simulink model "InnerOuter_Sim"  (Simulink 6.6)
settings: Solver=ode4  StartTime=0.0  StopTime=700  FixedStep=SampleT  RelTol=1e-3
InitFcn:
  | clc
  | Rascal_Var
  | innerOuterInit
  | wpFile
values from neighbouring files (symbols this model uses):
  A1 = 0.007    [Rascal_Var.m]
  Apolar = 0.057    [Rascal_Var.m]
  apSampleTime = 0.01    [innerOuterInit.m]
  CD0 = 0.022    [Rascal_Var.m]
  chord = S/span    (= 0.351341681574)    [Rascal_Var.m]
  CL0 = 0.38    [Rascal_Var.m]
  CLa = 18.5    [Rascal_Var.m]
  CLa_dot = 2.64    [Rascal_Var.m]
  Clb = -0.296    [Rascal_Var.m]
  ClDa = 0.1695    [Rascal_Var.m]
  CLDe = 0.24    [Rascal_Var.m]
  CLDf = 0.4    [Rascal_Var.m]
  ClDr = 0.106    [Rascal_Var.m]
  Clp = -1.96    [Rascal_Var.m]
  CLq = 7.4    [Rascal_Var.m]
  Clr = 0.103    [Rascal_Var.m]
  Cm0 = 0.3    [Rascal_Var.m]
  Cma = -1.239    [Rascal_Var.m]
  CmDe = -3.2    [Rascal_Var.m]
  CmDf = -.021    (= -0.021)    [Rascal_Var.m]
  Cmq = -2.4    [Rascal_Var.m]
  Cnb = 0.277    [Rascal_Var.m]
  CnDa = -0.023    [Rascal_Var.m]
  CnDr = -0.1997    [Rascal_Var.m]
  Cnp = -0.0889    [Rascal_Var.m]
  Cnr = -0.19997    [Rascal_Var.m]
  CYb = -1.098    [Rascal_Var.m]
  CYDr = 0.143    [Rascal_Var.m]
  derivativesConstant = 5    [innerOuterInit.m]
  elarm = 1.21    [Rascal_Var.m]
  Euler_0 = [0; 0; 90*pi/180]'    [Rascal_Var.m]    (also in randomInit.m = double([0; 0; psi_ic]'))
  ISA_g = 9.815    [Rascal_Var.m]
  Ixx = 4.12    [Rascal_Var.m]
  Iyy = 9.58    [Rascal_Var.m]
  Izz = 9.85    [Rascal_Var.m]
  mass = 0.45359237*18    (= 8.16466266)    [Rascal_Var.m]
  MinThK = 0.077    [Rascal_Var.m]
  Pos_0 = [0; 0 ;450]'    [Rascal_Var.m]    (also in randomInit.m = double([x_ic y_ic z_ic]))
  PQR_0 = [0;0;0]'    [Rascal_Var.m]
  SampleT = 0.005    [Rascal_Var.m]    (also in innerOuterInit.m)
  span = 2.795    [Rascal_Var.m]
  ThK = 2.17    [Rascal_Var.m]
  Vb_0 = [ 25; 0;0]'    [Rascal_Var.m]
  wpCount = uint8(floor(getRanVal(7,4,10)))    [randomInit.m]
undefined symbols (not defined in the file or in its folder): bankCommandLimit, clock, daLimit, deg, deLimit, DiscIntNeverNeededParam, drLimit, dtLimit, Earth, heightErrorLimit, pitchCommandLimit, pitchErrorLimit, rad, rollControlLimit, s, uHoldLimit, WGS84, yawDamperLimit
libraries: simulink x54, SLUGS_Library x14, aerolibconvert2 x9, aerolibtransform2 x2, aerolibwind2 x1, aerolibatmos2 x1, dspmtrx3 x1, dsPICdrivers x1
(part 1 of 2)
CloseFcn:
  | rtwprivate ssgencode ModelCloseRequest AttitudeComplementary
settings Model: Creator=ASL_Lab  LastModifiedBy=Administrator
settings DebuggingCC: ConsistencyChecking=warning  AlgebraicLoopMsg=error  MultiTaskDSMMsg=warning  MultiTaskCondExecSysMsg=none  ModelReferenceExtraNoncontSigs=warning  StrictBusMsg=None
settings HardwareCC: TargetHWDeviceType=32-bit Generic
settings RTWCC: IncludeERTFirstTime=on

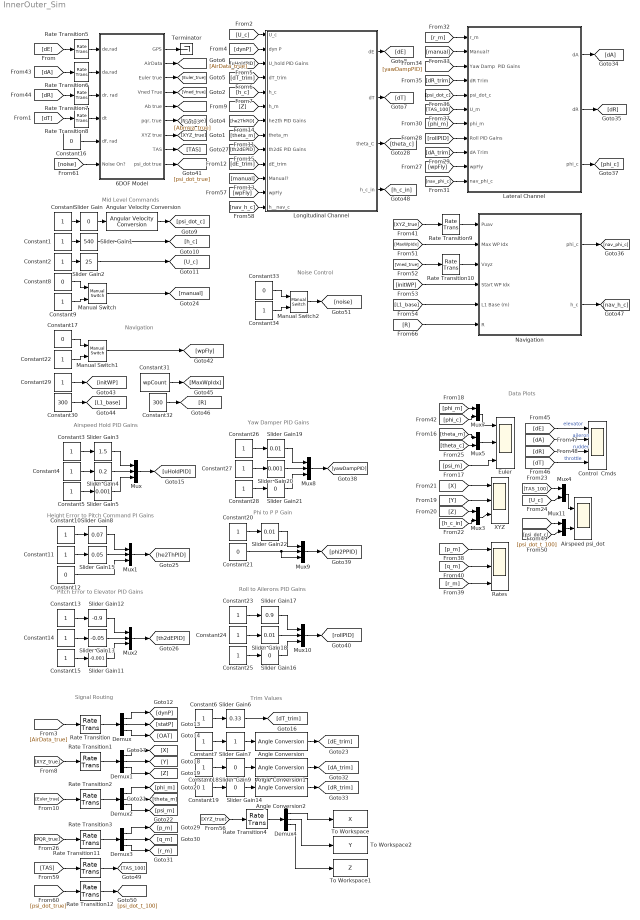
== system InnerOuter_Sim ==
  note: Mid Level Commands
  note: Trim Values
  note: Signal Routing
  note: Airspeed Hold PID Gains
  note: Height Error to Pitch Command PI Gains
  note: Pitch Error to Elevator PID Gains
  note: Data Plots
  note: Yaw Damper PID Gains
  note: Phi to P P Gain
  note: Roll to Ailerons PID Gains
  note: Navigation
  note: Noise Control
  6DOF Model : Subsystem
  Airspeed psi_dot : Scope  NumInputPorts=2
      settings: TimeRange=300  YMin=22.5~-0.3  YMax=37.5~0.25  SaveName=AirspeedPsiDot
  Angle Conversion : aerolibconvert2/Angle Conversion  SystemSampleTime=-1  IU=deg  OU=rad
  Angle Conversion1 : aerolibconvert2/Angle Conversion  SystemSampleTime=-1  IU=deg  OU=rad
  Angle Conversion2 : aerolibconvert2/Angle Conversion  SystemSampleTime=-1  IU=deg  OU=rad
  Angular Velocity Conversion : aerolibconvert2/Angular Velocity Conversion  SystemSampleTime=-1  IU=deg/s  OU=rad/s
  Constant{,1..7,9..11,13..15,18..20,22..29} (25 alike) : Constant  SampleTime=apSampleTime
  Constant{8,12,17,21} (4 alike) : Constant  Value=0  SampleTime=apSampleTime
  Constant16 : Constant  Value=0
  Constant30 : Constant  Value=300  SampleTime=apSampleTime
  Constant31 : Constant  Value=wpCount  SampleTime=apSampleTime
  Constant32 : Constant  Value=300  SampleTime=apSampleTime
  Constant33 : Constant  Value=0  SampleTime=SampleT
  Constant34 : Constant  SampleTime=SampleT
  Control  Cmds : Scope  NumInputPorts=4
      settings: TickLabels=on  TimeRange=300  YMin=-0.15~-0.075~-0.0015~0.4  YMax=0.15~0.1~0.002~0.9  SaveName=ScopeData12
  Demux{,1..4} (5 alike) : Demux  Outputs=3
  Euler : Scope  NumInputPorts=3
      settings: TimeRange=300  YMin=-0.35~-0.3~-0.5  YMax=0.7~0.3~6.5  SaveName=EulerData  DataFormat=Structure
  Lateral Channel : Subsystem  TreatAsAtomicUnit=on
  Longitudinal Channel : Subsystem  TreatAsAtomicUnit=on
  Manual Switch : simulink/Signal Routing/Manual Switch  SystemSampleTime=-1  sw=1  action=0  varsize=off
  Manual Switch1 : simulink/Signal Routing/Manual Switch  SystemSampleTime=-1  sw=0  action=0  varsize=off
  Manual Switch2 : simulink/Signal Routing/Manual Switch  SystemSampleTime=-1  sw=0  action=0  varsize=off
  Mux{,1..2,8..10} (6 alike) : Mux  Inputs=3
  Mux{3..5,7,11} (5 alike) : Mux  Inputs=2
  Navigation : Subsystem  TreatAsAtomicUnit=on
  Rate Transition{,1..4,9..12} (9 alike) : RateTransition  OutPortSampleTime=apSampleTime
  Rate Transition{5..8} (4 alike) : RateTransition  OutPortSampleTime=SampleT
  Rates : Scope  NumInputPorts=3
      settings: TimeRange=300  YMin=-0.75~-1.5~-0.3  YMax=1~1.5~0.7  SaveName=ScopeData3
  Slider Gain : simulink/Math Operations/Slider Gain  SystemSampleTime=-1  low=-20  gain=0  high=20
  Slider Gain1 : simulink/Math Operations/Slider Gain  SystemSampleTime=-1  low=0  gain=540  high=800
  Slider Gain11 : simulink/Math Operations/Slider Gain  SystemSampleTime=-1  low=-0.1  gain=-0.001  high=0
  Slider Gain12 : simulink/Math Operations/Slider Gain  SystemSampleTime=-1  low=-0.9  gain=-0.9  high=0.3
  Slider Gain13 : simulink/Math Operations/Slider Gain  SystemSampleTime=-1  low=-0.05  gain=-0.05  high=0
  Slider Gain14 : simulink/Math Operations/Slider Gain  SystemSampleTime=-1  low=-10  gain=0  high=10
  Slider Gain15 : simulink/Math Operations/Slider Gain  SystemSampleTime=-1  low=-20  gain=0.05  high=20
  Slider Gain16 : simulink/Math Operations/Slider Gain  SystemSampleTime=-1  low=-0.1  gain=0  high=0
  Slider Gain17 : simulink/Math Operations/Slider Gain  SystemSampleTime=-1  low=-0.1  gain=0.9  high=5
  Slider Gain18 : simulink/Math Operations/Slider Gain  SystemSampleTime=-1  low=-0.01  gain=0.01  high=0.01
  Slider Gain19 : simulink/Math Operations/Slider Gain  SystemSampleTime=-1  low=-20  gain=0.01  high=20
  Slider Gain2 : simulink/Math Operations/Slider Gain  SystemSampleTime=-1  low=1  gain=25  high=40
  Slider Gain20 : simulink/Math Operations/Slider Gain  SystemSampleTime=-1  low=-20  gain=0.001  high=20
  Slider Gain21 : simulink/Math Operations/Slider Gain  SystemSampleTime=-1  low=-20  gain=0  high=20
  Slider Gain22 : simulink/Math Operations/Slider Gain  SystemSampleTime=-1  low=-20  gain=0.01  high=20
  Slider Gain3 : simulink/Math Operations/Slider Gain  SystemSampleTime=-1  low=-20  gain=1.5  high=20
  Slider Gain4 : simulink/Math Operations/Slider Gain  SystemSampleTime=-1  low=-20  gain=0.2  high=20
  Slider Gain5 : simulink/Math Operations/Slider Gain  SystemSampleTime=-1  low=-20  gain=0.001  high=20
  Slider Gain6 : simulink/Math Operations/Slider Gain  SystemSampleTime=-1  low=0.1  gain=0.33  high=1
  Slider Gain7 : simulink/Math Operations/Slider Gain  SystemSampleTime=-1  low=-10  gain=1  high=10
  Slider Gain8 : simulink/Math Operations/Slider Gain  SystemSampleTime=-1  low=-20  gain=0.07  high=20
  Slider Gain9 : simulink/Math Operations/Slider Gain  SystemSampleTime=-1  low=-10  gain=0  high=10
  Terminator : Terminator
  To Workspace : ToWorkspace  VariableName=X  SampleTime=-1  SaveFormat=Array
  To Workspace1 : ToWorkspace  VariableName=Z  SampleTime=-1  SaveFormat=Array
  To Workspace2 : ToWorkspace  VariableName=Y  SampleTime=-1  SaveFormat=Array
  XYZ : Scope  NumInputPorts=3
      settings: TimeRange=300  YMin=0~-400~0  YMax=2500~700~800
  wires:
  6DOF Model/7(XYZ true) -> [XYZ_true]
  6DOF Model/4(Vned True) -> [Vned_true]
  6DOF Model/5(Ab true) -> [Abmea_true]
  6DOF Model/6("pqr, true") -> [PQR_true]
  6DOF Model/3(Euler true) -> [Euler_true]
  6DOF Model/2(AirData) -> [AirData_true]
  Longitudinal Channel/1(dE) -> [dE]
  Longitudinal Channel/2(dT) -> [dT]
  Constant/1 -> Slider Gain/1
  Constant1/1 -> Slider Gain1/1
  Constant2/1 -> Slider Gain2/1
  Slider Gain/1 -> Angular Velocity Conversion/1
  Angular Velocity Conversion/1 -> [psi_dot_c]
  Slider Gain2/1 -> [U_c]
  [U_c] -> Longitudinal Channel/1(U_c)
  [AirData_true] -> Rate Transition/1
  Demux/1 -> [dynP]
  Demux/2 -> [statP]
  Demux/3 -> [OAT]
  Constant3/1 -> Slider Gain3/1
  Constant4/1 -> Slider Gain4/1
  Constant5/1 -> Slider Gain5/1
  Slider Gain4/1 -> Mux/2
  Slider Gain3/1 -> Mux/1
  Slider Gain5/1 -> Mux/3
  Mux/1 -> [uHoldPID]
  [dynP] -> Longitudinal Channel/2(dyn P)
  [uHoldPID] -> Longitudinal Channel/3(U_hold PID Gains)
  Constant6/1 -> Slider Gain6/1
  Slider Gain6/1 -> [dT_trim]
  [dT_trim] -> Longitudinal Channel/4(dT_trim)
  [h_c] -> Longitudinal Channel/5(h_c)
  [XYZ_true] -> Rate Transition1/1
  Demux1/1 -> [X]
  Demux1/2 -> [Y]
  Demux1/3 -> [Z]
  [Z] -> Longitudinal Channel/6(h_m)
  [Euler_true] -> Rate Transition2/1
  Demux2/1 -> [phi_m]
  Demux2/2 -> [theta_m]
  Demux2/3 -> [psi_m]
  [theta_m] -> Longitudinal Channel/8(theta_m)
  Constant7/1 -> Slider Gain7/1
  Slider Gain7/1 -> Angle Conversion/1
  Angle Conversion/1 -> [dE_trim]
  [dE_trim] -> Longitudinal Channel/10(dE_trim)
  Constant8/1 -> Manual Switch/1
  Constant9/1 -> Manual Switch/2
  Manual Switch/1 -> [manual]
  [manual] -> Longitudinal Channel/11(Manual?)
  Constant10/1 -> Slider Gain8/1
  Constant11/1 -> Slider Gain15/1
  Constant12/1 -> Mux1/3
  Slider Gain8/1 -> Mux1/1
  Mux1/1 -> [he2ThPID]
  Constant13/1 -> Slider Gain12/1
  Constant14/1 -> Slider Gain13/1
  Constant15/1 -> Slider Gain11/1
  Slider Gain13/1 -> Mux2/2
  Slider Gain12/1 -> Mux2/1
  Slider Gain11/1 -> Mux2/3
  Mux2/1 -> [th2dEPID]
  [he2ThPID] -> Longitudinal Channel/7(he2th PID Gains)
  [th2dEPID] -> Longitudinal Channel/9(th2dE PID Gains)
  Mux5/1 -> Euler/2
  [psi_m] -> Euler/3
  [X] -> XYZ/1
  [Y] -> XYZ/2
  Mux3/1 -> XYZ/3
  [Z] -> Mux3/1
  [h_c_in] -> Mux3/2
  [dT] -> Rate Transition8/1
  [dE] -> Rate Transition5/1
  Mux4/1 -> Airspeed psi_dot/1
  6DOF Model/8(TAS) -> [TAS]
  [TAS_100] -> Mux4/1
  [U_c] -> Mux4/2
  [theta_c] -> Mux5/2
  Longitudinal Channel/3(theta_C) -> [theta_c]
  [PQR_true] -> Rate Transition3/1
  Demux3/1 -> [p_m]
  Demux3/2 -> [q_m]
  Demux3/3 -> [r_m]
  Constant18/1 -> Slider Gain9/1
  Slider Gain9/1 -> Angle Conversion1/1
  Angle Conversion1/1 -> [dA_trim]
  Constant19/1 -> Slider Gain14/1
  Slider Gain14/1 -> Angle Conversion2/1
  Angle Conversion2/1 -> [dR_trim]
  [r_m] -> Lateral Channel/1(r_m)
  [manual] -> Lateral Channel/2(Manual?)
  [yawDampPID] -> Lateral Channel/3(Yaw Damp  PID Gains)
  [dR_trim] -> Lateral Channel/4(dR Trim)
  [psi_dot_c] -> Lateral Channel/5(psi_dot_c)
  [TAS_100] -> Lateral Channel/6(U_m)
  [phi_m] -> Lateral Channel/7(phi_m)
  [rollPID] -> Lateral Channel/8(Roll PID Gains)
  [dA_trim] -> Lateral Channel/9(dA Trim)
  [r_m] -> Rates/3
  Lateral Channel/1(dA) -> [dA]
  Lateral Channel/2(dR) -> [dR]
  Lateral Channel/3(phi_c) -> [phi_c]
  [q_m] -> Rates/2
  [phi_m] -> Mux7/1
  [phi_c] -> Mux7/2
  Mux7/1 -> Euler/1
  Constant26/1 -> Slider Gain19/1
  Constant27/1 -> Slider Gain20/1
  Constant28/1 -> Slider Gain21/1
  Slider Gain20/1 -> Mux8/2
  Slider Gain19/1 -> Mux8/1
  Slider Gain21/1 -> Mux8/3
  Mux8/1 -> [yawDampPID]
  Constant20/1 -> Slider Gain22/1
  Constant21/1 -> Mux9/2, Mux9/3
  Slider Gain22/1 -> Mux9/1
  Mux9/1 -> [phi2PPID]
  Constant23/1 -> Slider Gain17/1
  Constant24/1 -> Slider Gain18/1
  Constant25/1 -> Slider Gain16/1
  Slider Gain18/1 -> Mux10/2
  Slider Gain17/1 -> Mux10/1
  Slider Gain16/1 -> Mux10/3
  Mux10/1 -> [rollPID]
  [dA] -> Rate Transition6/1
  [dR] -> Rate Transition7/1
  Constant16/1 -> 6DOF Model/5("df, rad")
  Slider Gain15/1 -> Mux1/2
  [dE] -> Control  Cmds/1  "elevator"
  [dA] -> Control  Cmds/2  "aileron"
  [dR] -> Control  Cmds/3  "rudder"
  [dT] -> Control  Cmds/4  "throttle"
  [theta_m] -> Mux5/1
  6DOF Model/9(psi_dot true) -> [psi_dot_true]
  [psi_dot_t_100] -> Mux11/1
  [psi_dot_c] -> Mux11/2
  Mux11/1 -> Airspeed psi_dot/2
  [p_m] -> Rates/1
  Constant17/1 -> Manual Switch1/1
  Constant22/1 -> Manual Switch1/2
  Manual Switch1/1 -> [wpFly]
  Constant29/1 -> [initWP]
  Slider Gain1/1 -> [h_c]
  [wpFly] -> Lateral Channel/10(wpFly)
  Navigation/1(phi_c) -> [nav_phi_c]
  [nav_phi_c] -> Lateral Channel/11(nav_phi_c)
  [XYZ_true] -> Rate Transition9/1
  Constant30/1 -> [L1_base]
  Constant31/1 -> [MaxWpIdx]
  [MaxWpIdx] -> Navigation/2(Max WP Idx)
  [Vned_true] -> Rate Transition10/1
  [initWP] -> Navigation/4(Start WP Idx)
  [L1_base] -> Navigation/5(L1 Base (m))
  [XYZ_true] -> Rate Transition4/1
  Demux4/1 -> To Workspace/1
  Demux4/2 -> To Workspace2/1
  Demux4/3 -> To Workspace1/1
  Navigation/2(h_c) -> [nav_h_c]
  [wpFly] -> Longitudinal Channel/12(wpFly)
  [nav_h_c] -> Longitudinal Channel/13(h__nav_c)
  Longitudinal Channel/4(h_c_in) -> [h_c_in]
  Rate Transition/1 -> Demux/1
  Rate Transition1/1 -> Demux1/1
  Rate Transition2/1 -> Demux2/1
  Rate Transition3/1 -> Demux3/1
  Rate Transition4/1 -> Demux4/1
  Rate Transition5/1 -> 6DOF Model/1(de,rad)
  Rate Transition6/1 -> 6DOF Model/2(da,rad)
  Rate Transition7/1 -> 6DOF Model/3("dr, rad")
  Rate Transition8/1 -> 6DOF Model/4(dt)
  Rate Transition9/1 -> Navigation/1(Puav)
  Rate Transition10/1 -> Navigation/3(Vxyz)
  [TAS] -> Rate Transition11/1
  Rate Transition11/1 -> [TAS_100]
  [psi_dot_true] -> Rate Transition12/1
  Rate Transition12/1 -> [psi_dot_t_100]
  Constant33/1 -> Manual Switch2/1
  Constant34/1 -> Manual Switch2/2
  Manual Switch2/1 -> [noise]
  [noise] -> 6DOF Model/6(Noise On?)
  Constant32/1 -> [R]
  [R] -> Navigation/6(R)
  6DOF Model/1(GPS) -> Terminator/1

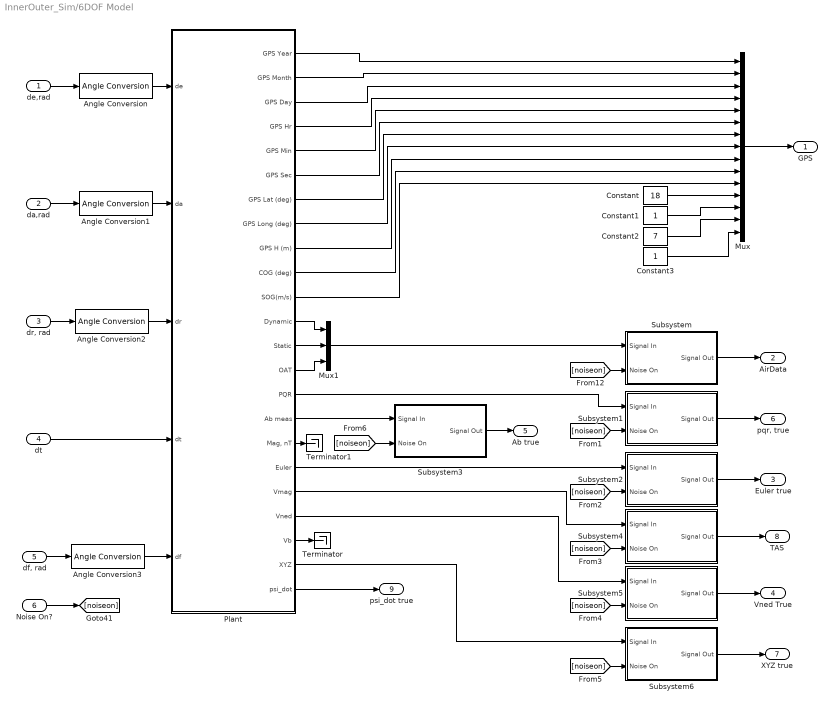
== system InnerOuter_Sim/6DOF Model ==
  de,rad : Inport
  da,rad : Inport  Port=2
  "dr, rad" : Inport  Port=3
  dt : Inport  Port=4
  "df, rad" : Inport  Port=5
  Noise On? : Inport  Port=6
  Angle Conversion{,1..3} (4 alike) : aerolibconvert2/Angle Conversion  SystemSampleTime=-1  IU=rad  OU=deg
  Constant : Constant  Value=18  SampleTime=SampleT
  Constant1 : Constant  SampleTime=SampleT
  Constant2 : Constant  Value=7  SampleTime=SampleT
  Constant3 : Constant  SampleTime=SampleT
  Mux : Mux  Inputs=15
  Mux1 : Mux  Inputs=3
  Plant : Subsystem
  Subsystem : Subsystem  mask{nv=[0.01 0.01 0.1], st=SampleT, ns=[132 564 987]}
      mask prompts: nv "Noise Variance"; st "Sample Time"; ns "Noise Seed"
  Subsystem1 : Subsystem  mask{nv=[0.001 0.001 0.001], st=SampleT, ns=[132 564 987]}
      mask prompts: nv "Noise Variance"; st "Sample Time"; ns "Noise Seed"
  Subsystem2 : Subsystem  mask{nv=[0.0001 0.00003 0.0001], st=SampleT, ns=[132 564 987]}
      mask prompts: nv "Noise Variance"; st "Sample Time"; ns "Noise Seed"
  Subsystem3 : Subsystem  mask{nv=[0.1 0.1 0.1], st=SampleT, ns=[132 564 987]}
      mask prompts: nv "Noise Variance"; st "Sample Time"; ns "Noise Seed"
  Subsystem4 : Subsystem  mask{nv=[0.01], st=SampleT, ns=[321564]}
      mask prompts: nv "Noise Variance"; st "Sample Time"; ns "Noise Seed"
  Subsystem5 : Subsystem  mask{nv=[0.01 0.01 0.01], st=SampleT, ns=[321564 6546 98798]}
      mask prompts: nv "Noise Variance"; st "Sample Time"; ns "Noise Seed"
  Subsystem6 : Subsystem  mask{nv=[0.03 0.03 0.05], st=SampleT, ns=[321564]}
      mask prompts: nv "Noise Variance"; st "Sample Time"; ns "Noise Seed"
  Terminator : Terminator
  Terminator1 : Terminator
  GPS : Outport
  AirData : Outport  Port=2
  Euler true : Outport  Port=3
  Vned True : Outport  Port=4
  Ab true : Outport  Port=5
  "pqr, true" : Outport  Port=6
  XYZ true : Outport  Port=7
  TAS : Outport  Port=8
  psi_dot true : Outport  Port=9
  wires:
  de,rad/1 -> Angle Conversion/1
  da,rad/1 -> Angle Conversion1/1
  "dr, rad"/1 -> Angle Conversion2/1
  dt/1 -> Plant/4(dt)
  "df, rad"/1 -> Angle Conversion3/1
  Angle Conversion/1 -> Plant/1(de)
  Angle Conversion1/1 -> Plant/2(da)
  Angle Conversion2/1 -> Plant/3(dr)
  Angle Conversion3/1 -> Plant/5(df)
  Mux/1 -> GPS/1
  Plant/1(GPS Year) -> Mux/1
  Plant/2(GPS Month) -> Mux/2
  Plant/3(GPS Day) -> Mux/3
  Plant/4(GPS Hr) -> Mux/4
  Plant/5(GPS Min) -> Mux/5
  Plant/6(GPS Sec) -> Mux/6
  Plant/7(GPS Lat (deg)) -> Mux/7
  Plant/8(GPS Long (deg)) -> Mux/8
  Plant/9(GPS H (m)) -> Mux/9
  Plant/10(COG (deg)) -> Mux/10
  Plant/11(SOG(m/s)) -> Mux/11
  Plant/12(Dynamic) -> Mux1/1
  Plant/13(Static) -> Mux1/2
  Plant/14(OAT) -> Mux1/3
  Mux1/1 -> Subsystem/1(Signal In)
  Constant/1 -> Mux/12
  Constant1/1 -> Mux/13
  Constant2/1 -> Mux/14
  Constant3/1 -> Mux/15
  Plant/23(psi_dot) -> psi_dot true/1
  Noise On?/1 -> [noiseon]
  Subsystem/1(Signal Out) -> AirData/1
  [noiseon] -> Subsystem/2(Noise On)
  [noiseon] -> Subsystem1/2(Noise On)
  [noiseon] -> Subsystem2/2(Noise On)
  [noiseon] -> Subsystem4/2(Noise On)
  [noiseon] -> Subsystem5/2(Noise On)
  [noiseon] -> Subsystem6/2(Noise On)
  [noiseon] -> Subsystem3/2(Noise On)
  Subsystem1/1(Signal Out) -> "pqr, true"/1
  Plant/15(PQR) -> Subsystem1/1(Signal In)
  Subsystem2/1(Signal Out) -> Euler true/1
  Plant/18(Euler) -> Subsystem2/1(Signal In)
  Subsystem3/1(Signal Out) -> Ab true/1
  Plant/16(Ab meas) -> Subsystem3/1(Signal In)
  Subsystem4/1(Signal Out) -> TAS/1
  Plant/19(Vmag) -> Subsystem4/1(Signal In)
  Subsystem5/1(Signal Out) -> Vned True/1
  Plant/20(Vned) -> Subsystem5/1(Signal In)
  Subsystem6/1(Signal Out) -> XYZ true/1
  Plant/22(XYZ) -> Subsystem6/1(Signal In)
  Plant/21(Vb) -> Terminator/1
  Plant/17("Mag, nT") -> Terminator1/1

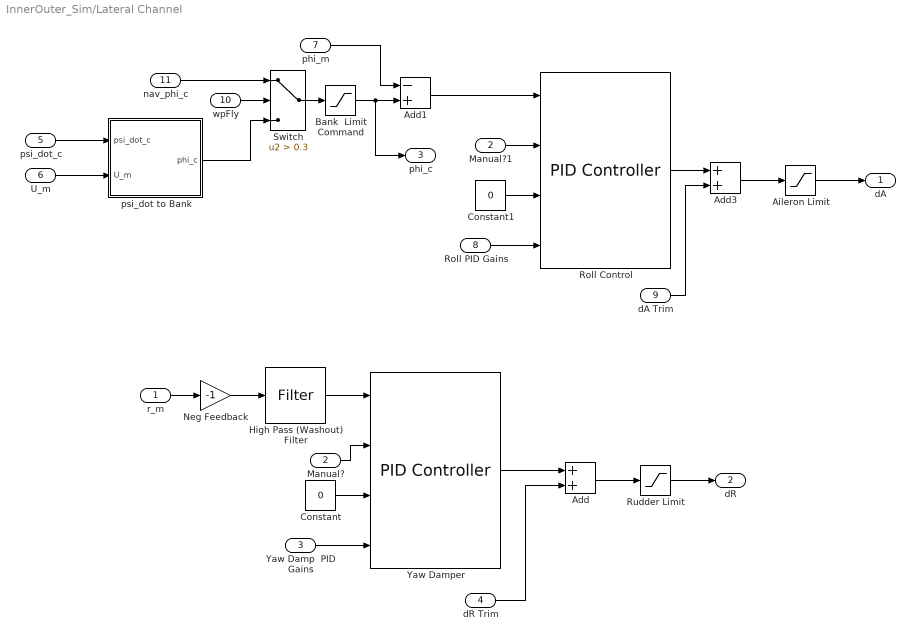
== system InnerOuter_Sim/Lateral Channel ==
  r_m : Inport
  Manual? : Inport  Port=2
  Yaw Damp  PID Gains : Inport  Port=3
  dR Trim : Inport  Port=4
  psi_dot_c : Inport  Port=5
  U_m : Inport  Port=6
  phi_m : Inport  Port=7
  Roll PID Gains : Inport  Port=8
  dA Trim : Inport  Port=9
  wpFly : Inport  Port=10  SampleTime=apSampleTime
  nav_phi_c : Inport  Port=11
  Add : Sum  OutScaling=2^-10
  Add1 : Sum  Inputs=-+  OutScaling=2^-10
  Add3 : Sum  OutScaling=2^-10
  Aileron Limit : Saturate  UpperLimit=daLimit  LowerLimit=-daLimit  SampleTime=apSampleTime
  Bank  Limit Command : Saturate  UpperLimit=bankCommandLimit  LowerLimit=-bankCommandLimit  SampleTime=apSampleTime
  Constant : Constant  Value=0
  Constant1 : Constant  Value=0
  High Pass (Washout) Filter : SLUGS_Library/Singnal Routing & Conditioning/Filter  SystemSampleTime=-1  Zeros=[0]  Poles=[-1/5]  Gain=1  AbsTol=auto  SampleTime=apSampleTime  method=tustin  Wc=1
  Manual?1 : InportShadow  Port=2  LatchByCopyingInsideSignal=off
  Neg Feedback : Gain  Gain=-1
  Roll Control : SLUGS_Library/Control Blocks/PID Controller  SystemSampleTime=-1  TSample=apSampleTime  NDelay=derivativesConstant  upperLimit=rollControlLimit  lowerLimit=-rollControlLimit
  Rudder Limit : Saturate  UpperLimit=apSampleTime  LowerLimit=-drLimit  SampleTime=apSampleTime
  Switch : Switch  Criteria=u2 > Threshold  Threshold=0.3
  Yaw Damper : SLUGS_Library/Control Blocks/PID Controller  SystemSampleTime=-1  TSample=apSampleTime  NDelay=derivativesConstant  upperLimit=yawDamperLimit  lowerLimit=-yawDamperLimit
  psi_dot to Bank : Subsystem
  dA : Outport
  dR : Outport  Port=2
  phi_c : Outport  Port=3
  wires:
  High Pass (Washout) Filter/1 -> Yaw Damper/1
  Neg Feedback/1 -> High Pass (Washout) Filter/1
  r_m/1 -> Neg Feedback/1
  Rudder Limit/1 -> dR/1
  Constant/1 -> Yaw Damper/3
  Manual?/1 -> Yaw Damper/2
  Yaw Damp  PID Gains/1 -> Yaw Damper/4
  Add/1 -> Rudder Limit/1
  Yaw Damper/1 -> Add/1
  dR Trim/1 -> Add/2
  psi_dot_c/1 -> psi_dot to Bank/1(psi_dot_c)
  U_m/1 -> psi_dot to Bank/2(U_m)
  Manual?1/1 -> Roll Control/2
  Constant1/1 -> Roll Control/3
  Roll PID Gains/1 -> Roll Control/4
  Add3/1 -> Aileron Limit/1
  Roll Control/1 -> Add3/1
  dA Trim/1 -> Add3/2
  Aileron Limit/1 -> dA/1
  Add1/1 -> Roll Control/1
  phi_m/1 -> Add1/1
  Switch/1 -> Bank  Limit Command/1
  nav_phi_c/1 -> Switch/1
  wpFly/1 -> Switch/2
  psi_dot to Bank/1(phi_c) -> Switch/3
  Bank  Limit Command/1 -> Add1/2, phi_c/1

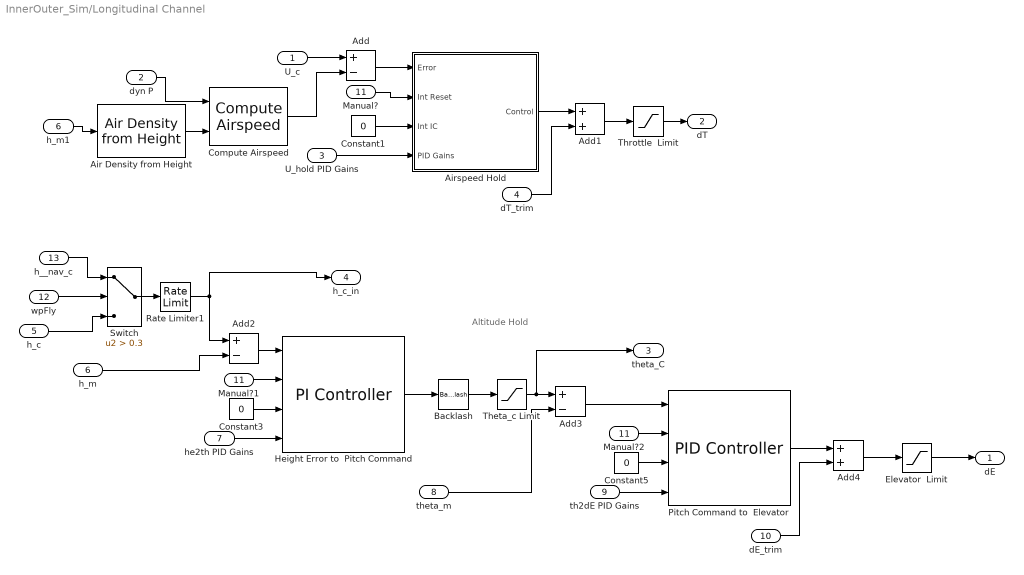
== system InnerOuter_Sim/Longitudinal Channel ==
  note: Altitude Hold
  U_c : Inport
  dyn P : Inport  Port=2
  U_hold PID Gains : Inport  Port=3
  dT_trim : Inport  Port=4
  h_c : Inport  Port=5
  h_m : Inport  Port=6
  he2th PID Gains : Inport  Port=7
  theta_m : Inport  Port=8
  th2dE PID Gains : Inport  Port=9
  dE_trim : Inport  Port=10
  Manual? : Inport  Port=11
  wpFly : Inport  Port=12  SampleTime=apSampleTime
  h__nav_c : Inport  Port=13
  Add : Sum  Inputs=+-  OutScaling=2^-10
  Add1 : Sum  Inputs=2  OutScaling=2^-10
  Add2 : Sum  Inputs=+-  OutScaling=2^-10
  Add3 : Sum  Inputs=+-  OutScaling=2^-10
  Add4 : Sum  Inputs=2  OutScaling=2^-10
  Air Density from Height : SLUGS_Library/Air Density from Height  SystemSampleTime=-1
  Airspeed Hold : Subsystem  AncestorBlock=SLUGS_Library/Control Blocks/PID Controller  mask{TSample=apSampleTime, NDelay=derivativesConstant, upperLimit=uHoldLimit, lowerLimit=0.1}
      mask prompts: TSample "Sample Time"; NDelay "Derivation Time Constant Factor (1->10)"; upperLimit "Integrator Upper Windup Limit"; lowerLimit "Integrator Lower Windup Limit"
      mask help:
      | This Block implements a PID Controller with the Following Characteristcs:
      |
      | 1.- Integrator antiwindup is given by the limits in the block
      | 2.- The time Derivative is "low-passed" by using the previous N samples instead of the one before
      | 3.- It contains an Integrator Reset if needed
  Backlash : Backlash  BacklashWidth=0.05
  Compute Airspeed : SLUGS_Library/Compute Airspeed  SystemSampleTime=-1
  Constant1 : Constant  Value=0
  Constant3 : Constant  Value=0
  Constant5 : Constant  Value=0
  Elevator  Limit : Saturate  UpperLimit=deLimit  LowerLimit=-deLimit  SampleTime=apSampleTime
  Height Error to  Pitch Command : SLUGS_Library/Control Blocks/PI Controller  SystemSampleTime=-1  TSample=apSampleTime  upperLimit=heightErrorLimit  lowerLimit=-heightErrorLimit
  Manual?1 : InportShadow  Port=11  LatchByCopyingInsideSignal=off
  Manual?2 : InportShadow  Port=11  LatchByCopyingInsideSignal=off
  Pitch Command to  Elevator : SLUGS_Library/Control Blocks/PID Controller  SystemSampleTime=-1  TSample=apSampleTime  NDelay=derivativesConstant  upperLimit=pitchErrorLimit  lowerLimit=-pitchErrorLimit
  Rate Limiter1 : RateLimiter  RisingSlewLimit=10  FallingSlewLimit=-10  SampleTimeMode=inherited
  Switch : Switch  Criteria=u2 > Threshold  Threshold=0.3
  Theta_c Limit : Saturate  UpperLimit=pitchCommandLimit  LowerLimit=-pitchCommandLimit  SampleTime=apSampleTime
  Throttle  Limit : Saturate  UpperLimit=dtLimit  LowerLimit=0  SampleTime=apSampleTime
  h_m1 : InportShadow  Port=6  LatchByCopyingInsideSignal=off
  dE : Outport
  dT : Outport  Port=2
  theta_C : Outport  Port=3
  h_c_in : Outport  Port=4
  wires:
  U_c/1 -> Add/1
  Compute Airspeed/1 -> Add/2
  Add/1 -> Airspeed Hold/1(Error)
  Airspeed Hold/1(Control) -> Add1/1
  dT_trim/1 -> Add1/2
  Add1/1 -> Throttle  Limit/1
  Constant1/1 -> Airspeed Hold/3(Int IC)
  U_hold PID Gains/1 -> Airspeed Hold/4(PID Gains)
  Throttle  Limit/1 -> dT/1
  Add2/1 -> Height Error to  Pitch Command/1
  h_m/1 -> Add2/2
  Constant3/1 -> Height Error to  Pitch Command/3
  theta_m/1 -> Add3/2
  Constant5/1 -> Pitch Command to  Elevator/3
  Manual?/1 -> Airspeed Hold/2(Int Reset)
  Manual?1/1 -> Height Error to  Pitch Command/2
  Manual?2/1 -> Pitch Command to  Elevator/2
  Add4/1 -> Elevator  Limit/1
  Pitch Command to  Elevator/1 -> Add4/1
  dE_trim/1 -> Add4/2
  Elevator  Limit/1 -> dE/1
  Air Density from Height/1 -> Compute Airspeed/2
  dyn P/1 -> Compute Airspeed/1
  h_m1/1 -> Air Density from Height/1
  he2th PID Gains/1 -> Height Error to  Pitch Command/4
  th2dE PID Gains/1 -> Pitch Command to  Elevator/4
  Add3/1 -> Pitch Command to  Elevator/1
  Theta_c Limit/1 -> Add3/1, theta_C/1
  wpFly/1 -> Switch/2
  Switch/1 -> Rate Limiter1/1
  h_c/1 -> Switch/3
  h__nav_c/1 -> Switch/1
  Rate Limiter1/1 -> Add2/1, h_c_in/1
  Height Error to  Pitch Command/1 -> Backlash/1
  Backlash/1 -> Theta_c Limit/1

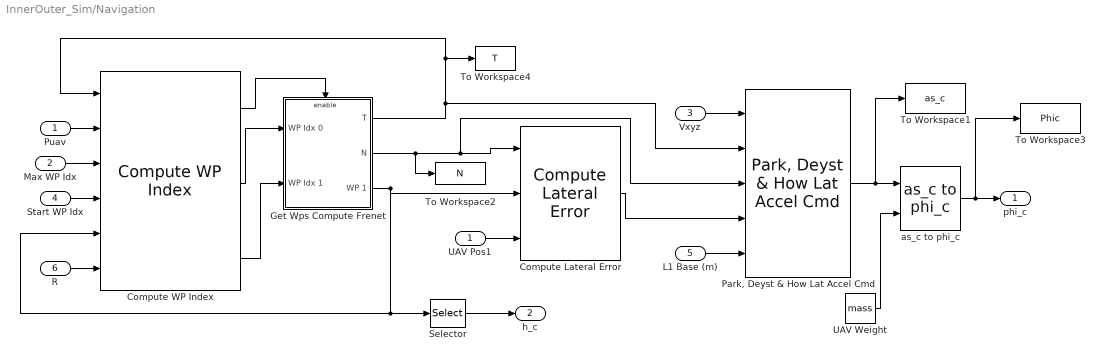
== system InnerOuter_Sim/Navigation ==
  Puav : Inport  SampleTime=apSampleTime
  Max WP Idx : Inport  Port=2
  Vxyz : Inport  Port=3
  Start WP Idx : Inport  Port=4
  L1 Base (m) : Inport  Port=5
  R : Inport  Port=6
  Compute Lateral Error : SLUGS_Library/Navigation/Compute Lateral Error  SystemSampleTime=-1
  Compute WP Index : SLUGS_Library/Navigation/Compute WP Index  SystemSampleTime=-1
  Get Wps Compute Frenet : Subsystem
  "Park, Deyst & How Lat Accel Cmd" : SLUGS_Library/Navigation/Park, Deyst & How Lat Accel Cmd  SystemSampleTime=-1
  Selector : Selector  IndexOptions=Index vector (dialog)  Indices=[3]  OutputSizes=1  InputPortWidth=3
  To Workspace1 : ToWorkspace  VariableName=as_c  SampleTime=-1  SaveFormat=Array
  To Workspace2 : ToWorkspace  VariableName=N  SampleTime=-1  SaveFormat=Array
  To Workspace3 : ToWorkspace  VariableName=Phic  SampleTime=-1  SaveFormat=Array
  To Workspace4 : ToWorkspace  VariableName=T  SampleTime=-1  SaveFormat=Array
  UAV Weight : Constant  Value=mass
  UAV Pos1 : InportShadow  Port=1  SampleTime=apSampleTime  LatchByCopyingInsideSignal=off
  as_c to phi_c : SLUGS_Library/Navigation/as_c to phi_c  SystemSampleTime=-1
  phi_c : Outport
  h_c : Outport  Port=2
  wires:
  Compute WP Index/2 -> Get Wps Compute Frenet/1(WP Idx 0)
  Compute WP Index/3 -> Get Wps Compute Frenet/2(WP Idx 1)
  Get Wps Compute Frenet/2(N) -> Compute Lateral Error/1, "Park, Deyst & How Lat Accel Cmd"/3, To Workspace2/1
  Get Wps Compute Frenet/1(T) -> To Workspace4/1, Compute WP Index/1, "Park, Deyst & How Lat Accel Cmd"/2
  Puav/1 -> Compute WP Index/2
  Max WP Idx/1 -> Compute WP Index/3
  Start WP Idx/1 -> Compute WP Index/4
  "Park, Deyst & How Lat Accel Cmd"/1 -> as_c to phi_c/1, To Workspace1/1
  UAV Pos1/1 -> Compute Lateral Error/3
  as_c to phi_c/1 -> phi_c/1, To Workspace3/1
  UAV Weight/1 -> as_c to phi_c/2
  Compute Lateral Error/1 -> "Park, Deyst & How Lat Accel Cmd"/4
  Get Wps Compute Frenet/3(WP 1) -> Compute Lateral Error/2, Selector/1, Compute WP Index/5
  Selector/1 -> h_c/1
  L1 Base (m)/1 -> "Park, Deyst & How Lat Accel Cmd"/5
  Compute WP Index/1 -> Get Wps Compute Frenet/Enable
  R/1 -> Compute WP Index/6
  Vxyz/1 -> "Park, Deyst & How Lat Accel Cmd"/1

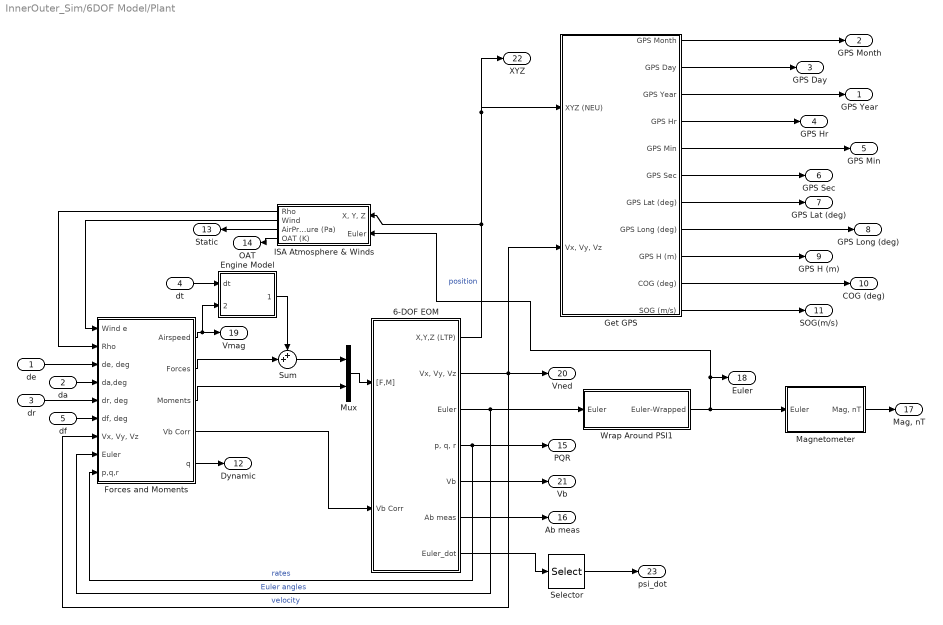
== system InnerOuter_Sim/6DOF Model/Plant ==
  de : Inport
  da : Inport  Port=2
  dr : Inport  Port=3
  dt : Inport  Port=4
  df : Inport  Port=5
  6-DOF EOM : Subsystem
  Engine Model : Subsystem
  Forces and Moments : Subsystem
  Get GPS : Subsystem
  ISA Atmosphere & Winds : Subsystem  Orientation=left
  Magnetometer : Subsystem  mask{magField=[ 23143.6 5858.2 45511.9]}
      mask prompts: magField "Local Magnetic Field"
      mask help:
      | Simulates the Data from magnetometers with no noise.
      |
      | You can obtain data for the local magnetic field at:
      |
      | http://www.ngdc.noaa.gov/geomagmodels/IGRFWMM.jsp
  Mux : Mux  Inputs=2
  Selector : Selector  IndexOptions=Index vector (dialog)  Indices=[3]  OutputSizes=1  InputPortWidth=3
  Sum : Sum  Inputs=++|  SaturateOnIntegerOverflow=on
  Wrap Around PSI1 : Subsystem
  GPS Year : Outport
  GPS Month : Outport  Port=2
  GPS Day : Outport  Port=3
  GPS Hr : Outport  Port=4
  GPS Min : Outport  Port=5
  GPS Sec : Outport  Port=6
  GPS Lat (deg) : Outport  Port=7
  GPS Long (deg) : Outport  Port=8
  GPS H (m) : Outport  Port=9
  COG (deg) : Outport  Port=10
  SOG(m/s) : Outport  Port=11
  Dynamic : Outport  Port=12
  Static : Outport  Orientation=left  Port=13
  OAT : Outport  Orientation=left  Port=14
  PQR : Outport  Port=15
  Ab meas : Outport  Port=16
  "Mag, nT" : Outport  Port=17
  Euler : Outport  Port=18
  Vmag : Outport  Port=19
  Vned : Outport  Port=20
  Vb : Outport  Port=21
  XYZ : Outport  Port=22
  psi_dot : Outport  Port=23
  wires:
  Get GPS/1(GPS Month) -> GPS Month/1
  Get GPS/2(GPS Day) -> GPS Day/1
  Get GPS/3(GPS Year) -> GPS Year/1
  Get GPS/4(GPS Hr) -> GPS Hr/1
  Get GPS/5(GPS Min) -> GPS Min/1
  Get GPS/6(GPS Sec) -> GPS Sec/1
  Get GPS/7(GPS Lat (deg)) -> GPS Lat (deg)/1
  Get GPS/8(GPS Long (deg)) -> GPS Long (deg)/1
  Get GPS/9(GPS H (m)) -> GPS H (m)/1
  6-DOF EOM/6(Ab meas) -> Ab meas/1
  Mux/1 -> 6-DOF EOM/1("[F,M]")
  6-DOF EOM/5(Vb) -> Vb/1
  Engine Model/1(Thrust) -> Sum/1
  Forces and Moments/5(q) -> Dynamic/1
  ISA Atmosphere & Winds/3(AirPressure (Pa)) -> Static/1
  Forces and Moments/1(Airspeed) -> Engine Model/2(Vmag), Vmag/1
  ISA Atmosphere & Winds/2(Wind) -> Forces and Moments/1(Wind e)
  ISA Atmosphere & Winds/1(Rho) -> Forces and Moments/2(Rho)
  Forces and Moments/3(Moments) -> Mux/2
  Forces and Moments/2(Forces) -> Sum/2
  Sum/1 -> Mux/1
  Forces and Moments/4(Vb Corr) -> 6-DOF EOM/2(Vb Corr)
  6-DOF EOM/1(X,Y,Z (LTP)) -> ISA Atmosphere & Winds/1("X, Y, Z"), Get GPS/1(XYZ (NEU)), XYZ/1  "position"
  6-DOF EOM/2("Vx, Vy, Vz") -> Vned/1, Get GPS/2("Vx, Vy, Vz"), Forces and Moments/7("Vx, Vy, Vz ")  "velocity"
  6-DOF EOM/3(Euler) -> Wrap Around PSI1/1(Euler), Forces and Moments/8(Euler)  "Euler angles"
  6-DOF EOM/4("p, q, r") -> PQR/1, Forces and Moments/9(p,q,r)  "rates"
  dt/1 -> Engine Model/1(dt)
  de/1 -> Forces and Moments/3("de, deg")
  da/1 -> Forces and Moments/4(da,deg)
  dr/1 -> Forces and Moments/5("dr, deg")
  df/1 -> Forces and Moments/6("df, deg")
  Wrap Around PSI1/1(Euler-Wrapped) -> Magnetometer/1(Euler), Euler/1, ISA Atmosphere & Winds/2(Euler)
  Magnetometer/1("Mag, nT") -> "Mag, nT"/1
  Get GPS/10(COG (deg)) -> COG (deg)/1
  Get GPS/11(SOG (m/s)) -> SOG(m/s)/1
  ISA Atmosphere & Winds/4(OAT (K)) -> OAT/1
  6-DOF EOM/7(Euler_dot) -> Selector/1
  Selector/1 -> psi_dot/1

== system InnerOuter_Sim/6DOF Model/Subsystem ==
  Signal In : Inport  Orientation=down
  Noise On : Inport  Port=2
  Add : Sum  OutScaling=2^-10
  Random Number : RandomNumber  Variance=nv  Seed=ns  SampleTime=st
  Signal1 : InportShadow  Port=1  LatchByCopyingInsideSignal=off
  Switch : Switch  Threshold=0.3
  Signal Out : Outport
  wires:
  Random Number/1 -> Add/2
  Add/1 -> Switch/1
  Signal In/1 -> Add/1
  Noise On/1 -> Switch/2
  Switch/1 -> Signal Out/1
  Signal1/1 -> Switch/3

== system InnerOuter_Sim/6DOF Model/Subsystem1 ==
  Signal In : Inport  Orientation=down
  Noise On : Inport  Port=2
  Add : Sum  OutScaling=2^-10
  Random Number : RandomNumber  Variance=nv  Seed=ns  SampleTime=st
  Signal1 : InportShadow  Port=1  LatchByCopyingInsideSignal=off
  Switch : Switch  Threshold=0.3
  Signal Out : Outport
  wires:
  Signal1/1 -> Switch/3
  Switch/1 -> Signal Out/1
  Noise On/1 -> Switch/2
  Signal In/1 -> Add/1
  Add/1 -> Switch/1
  Random Number/1 -> Add/2

== system InnerOuter_Sim/6DOF Model/Subsystem2 ==
  Signal In : Inport  Orientation=down
  Noise On : Inport  Port=2
  Add : Sum  OutScaling=2^-10
  Random Number : RandomNumber  Variance=nv  Seed=ns  SampleTime=st
  Signal1 : InportShadow  Port=1  LatchByCopyingInsideSignal=off
  Switch : Switch  Threshold=0.3
  Signal Out : Outport
  wires:
  Random Number/1 -> Add/2
  Add/1 -> Switch/1
  Signal In/1 -> Add/1
  Noise On/1 -> Switch/2
  Switch/1 -> Signal Out/1
  Signal1/1 -> Switch/3

== system InnerOuter_Sim/6DOF Model/Subsystem3 ==
  Signal In : Inport  Orientation=down
  Noise On : Inport  Port=2
  Add : Sum  OutScaling=2^-10
  Random Number : RandomNumber  Variance=nv  Seed=ns  SampleTime=st
  Signal1 : InportShadow  Port=1  LatchByCopyingInsideSignal=off
  Switch : Switch  Threshold=0.3
  Signal Out : Outport
  wires:
  Signal1/1 -> Switch/3
  Switch/1 -> Signal Out/1
  Noise On/1 -> Switch/2
  Signal In/1 -> Add/1
  Add/1 -> Switch/1
  Random Number/1 -> Add/2

== system InnerOuter_Sim/6DOF Model/Subsystem4 ==
  Signal In : Inport  Orientation=down
  Noise On : Inport  Port=2
  Add : Sum  OutScaling=2^-10
  Random Number : RandomNumber  Variance=nv  Seed=ns  SampleTime=st
  Signal1 : InportShadow  Port=1  LatchByCopyingInsideSignal=off
  Switch : Switch  Threshold=0.3
  Signal Out : Outport
  wires:
  Signal1/1 -> Switch/3
  Switch/1 -> Signal Out/1
  Noise On/1 -> Switch/2
  Signal In/1 -> Add/1
  Add/1 -> Switch/1
  Random Number/1 -> Add/2

== system InnerOuter_Sim/6DOF Model/Subsystem5 ==
  Signal In : Inport  Orientation=down
  Noise On : Inport  Port=2
  Add : Sum  OutScaling=2^-10
  Random Number : RandomNumber  Variance=nv  Seed=ns  SampleTime=st
  Signal1 : InportShadow  Port=1  LatchByCopyingInsideSignal=off
  Switch : Switch  Threshold=0.3
  Signal Out : Outport
  wires:
  Random Number/1 -> Add/2
  Add/1 -> Switch/1
  Signal In/1 -> Add/1
  Noise On/1 -> Switch/2
  Switch/1 -> Signal Out/1
  Signal1/1 -> Switch/3

== system InnerOuter_Sim/6DOF Model/Subsystem6 ==
  Signal In : Inport  Orientation=down
  Noise On : Inport  Port=2
  Add : Sum  OutScaling=2^-10
  Random Number : RandomNumber  Variance=nv  Seed=ns  SampleTime=st
  Signal1 : InportShadow  Port=1  LatchByCopyingInsideSignal=off
  Switch : Switch  Threshold=0.3
  Signal Out : Outport
  wires:
  Signal1/1 -> Switch/3
  Switch/1 -> Signal Out/1
  Noise On/1 -> Switch/2
  Signal In/1 -> Add/1
  Add/1 -> Switch/1
  Random Number/1 -> Add/2

== system InnerOuter_Sim/Lateral Channel/psi_dot to Bank ==
  psi_dot_c : Inport
  U_m : Inport  Port=2
  Constant1 : Constant  Value=9.80665
  Divide : Product  Inputs=**/  OutScaling=2^-10
  Subsystem : Subsystem
  phi_c : Outport
  wires:
  psi_dot_c/1 -> Divide/1
  U_m/1 -> Divide/2
  Constant1/1 -> Divide/3
  Subsystem/1(atan(x)) -> phi_c/1
  Divide/1 -> Subsystem/1(x)

== system InnerOuter_Sim/Longitudinal Channel/Airspeed Hold ==
  note: This Block implements a PID Controller with the
      | Following Characteristcs:
      | 1.- Antiwindup is given by the Limits in the block
      | 2.- The time Derivative is "low-passed" by using the
      | previous N samples instead of the one before
      | 3.- It contains an Integrator Reset if needed
  Error : Inport
  Int Reset : Inport  Port=2
  Int IC : Inport  Port=3
  PID Gains : Inport  Port=4
  Add : Sum  Inputs=3  OutScaling=2^-10
  Demux : Demux  Outputs=3
  Discrete-Time Integrator : DiscreteIntegrator  IntegratorMethod=Integration: Trapezoidal  ExternalReset=sampled level  InitialConditionSource=external  SampleTime=TSample  LimitOutput=on  UpperSaturationLimit=upperLimit  LowerSaturationLimit=lowerLimit  ICPrevOutput=DiscIntNeverNeededParam  ICPrevScaledInput=DiscIntNeverNeededParam
  Divide : Product  OutScaling=2^-10
  Divide1 : Product  OutScaling=2^-10
  Divide2 : Product  OutScaling=2^-10
  Low_passed Time Derivative : Subsystem
  Control : Outport
  wires:
  Divide2/1 -> Add/3
  Divide1/1 -> Add/2
  Demux/3 -> Divide2/1
  Demux/2 -> Divide1/1
  Add/1 -> Control/1
  Divide/1 -> Add/1
  Demux/1 -> Divide/1
  PID Gains/1 -> Demux/1
  Int IC/1 -> Discrete-Time Integrator/3
  Discrete-Time Integrator/1 -> Divide1/2
  Int Reset/1 -> Discrete-Time Integrator/2
  Error/1 -> Low_passed Time Derivative/1(f(t)), Divide/2, Discrete-Time Integrator/1
  Low_passed Time Derivative/1(f_dot(t)) -> Divide2/2

== system InnerOuter_Sim/Navigation/Get Wps Compute Frenet ==
  WP Idx 0 : Inport
  WP Idx 1 : Inport  Port=2
  Enable : EnablePort
  Compute Frenet : SLUGS_Library/Navigation/Compute Frenet  SystemSampleTime=-1
  get WP Coord from Index : SLUGS_Library/Navigation/get WP Coord from Index  SystemSampleTime=-1
  "get WP Coord from Index " : SLUGS_Library/Navigation/get WP Coord from Index  SystemSampleTime=-1
  T : Outport
  N : Outport  Port=2
  WP 1 : Outport  Port=3
  wires:
  "get WP Coord from Index "/1 -> WP 1/1, Compute Frenet/2
  get WP Coord from Index/1 -> Compute Frenet/1
  WP Idx 0/1 -> get WP Coord from Index/1
  Compute Frenet/1 -> T/1
  Compute Frenet/2 -> N/1
  WP Idx 1/1 -> "get WP Coord from Index "/1

== system InnerOuter_Sim/6DOF Model/Plant/6-DOF EOM ==
  "[F,M]" : Inport
  Vb Corr : Inport  Orientation=left  Port=2
  Angular Rates : Integrator  InitialCondition=PQR_0'
  Demux1 : Demux  Outputs=2
  Euler Angles : Integrator  InitialCondition=Euler_0
  Get Euler Dot : Subsystem
      mask Display:
      | port_label('input', 1, 'p, q, r')
      | port_label('input', 2, 'Euler')
      | port_label('output', 1, 'Euler_dot')
  Mux : Mux  Orientation=left  Inputs=[3;3]
  NED2NEU : Gain  Gain=[1 0 0;0 1 0;0 0 -1]  Multiplication=Matrix(K*u)  SaturateOnIntegerOverflow=on
  Position : Integrator  InitialCondition=Pos_0'
  RB2L * Vb : Product  Multiplication=Matrix(*)  SaturateOnIntegerOverflow=on  InputSameDT=on
  RB2LTP : Subsystem
  Velocities Body : Integrator  InitialCondition=Vb_0'
  "[V1,2,3,W1,2,3]" : Subsystem
  X,Y,Z (LTP) : Outport
  "Vx, Vy, Vz" : Outport  Port=2
  Euler : Outport  Port=3
  "p, q, r" : Outport  Orientation=left  Port=4
  Vb : Outport  Port=5
  Ab meas : Outport  Port=6
  Euler_dot : Outport  Port=7
  wires:
  "[V1,2,3,W1,2,3]"/1("Acc_meas ") -> Ab meas/1
  Euler Angles/1 -> "[V1,2,3,W1,2,3]"/2(Euler), Get Euler Dot/2(Euler), Euler/1, RB2LTP/1(Euler)
  Demux1/1 -> Velocities Body/1
  "[V1,2,3,W1,2,3]"/2(V*dot) -> Demux1/1
  Demux1/2 -> Angular Rates/1
  "[F,M]"/1 -> "[V1,2,3,W1,2,3]"/1("[F ; M]")
  RB2LTP/1(Rot) -> RB2L * Vb/1
  Velocities Body/1 -> Vb/1, RB2L * Vb/2
  Mux/1 -> "[V1,2,3,W1,2,3]"/3(V*)
  Position/1 -> X,Y,Z (LTP)/1
  Angular Rates/1 -> Get Euler Dot/1(p,q,r), Mux/2, "p, q, r"/1
  RB2L * Vb/1 -> NED2NEU/1, "Vx, Vy, Vz"/1  "NED"
  NED2NEU/1 -> Position/1
  Get Euler Dot/1(Euler_dot) -> Euler Angles/1, Euler_dot/1
  Vb Corr/1 -> Mux/1

== system InnerOuter_Sim/6DOF Model/Plant/Engine Model ==
  dt : Inport
  Vmag : Inport  Port=2
  Constant4 : Constant  Value=0
  Get To1 : Subsystem
  Mux : Mux  Inputs=2
  Mux1 : Mux  Inputs=3
  Thrust Available (lbs) : Fcn  Expr=u(1) - 0.047*sqrt(u(1))*u(2)
  kg2N : Gain  Gain=ISA_g  SaturateOnIntegerOverflow=on
  lbs2kg : Gain  Gain=0.45359237  SaturateOnIntegerOverflow=on
  Thrust : Outport
  wires:
  dt/1 -> Get To1/1(dt)
  Get To1/1(To) -> Mux/1
  Mux/1 -> Thrust Available (lbs)/1
  Thrust Available (lbs)/1 -> lbs2kg/1
  Vmag/1 -> Mux/2
  Mux1/1 -> Thrust/1
  lbs2kg/1 -> kg2N/1
  Constant4/1 -> Mux1/2, Mux1/3
  kg2N/1 -> Mux1/1

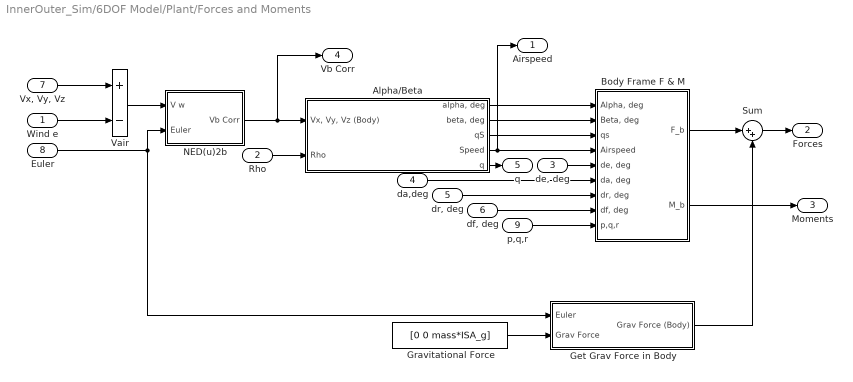
== system InnerOuter_Sim/6DOF Model/Plant/Forces and Moments ==
  Wind e : Inport
  Rho : Inport  Port=2
  "de, deg" : Inport  Port=3
  da,deg : Inport  Port=4
  "dr, deg" : Inport  Port=5
  "df, deg" : Inport  Port=6
  "Vx, Vy, Vz " : Inport  Port=7
  Euler : Inport  Port=8  PortDimensions=3
  p,q,r : Inport  Port=9
  Alpha/Beta : Subsystem
  Body Frame F & M : Subsystem
  Get Grav Force in Body : Subsystem
  Gravitational Force : Constant  Value=[0 0 mass*ISA_g]  VectorParams1D=off
  NED(u)2b : Subsystem
  Sum : Sum  Inputs=|++  SaturateOnIntegerOverflow=on
  Vair : Sum  Inputs=+-  SaturateOnIntegerOverflow=on  InputSameDT=on
  Airspeed : Outport
  Forces : Outport  Port=2
  Moments : Outport  Port=3
  Vb Corr : Outport  Port=4
  q : Outport  Port=5
  wires:
  Get Grav Force in Body/1(Grav Force (Body)) -> Sum/2
  Alpha/Beta/5(q) -> q/1
  "Vx, Vy, Vz "/1 -> Vair/1
  Vair/1 -> NED(u)2b/1(V w)
  Euler/1 -> NED(u)2b/2(Euler), Get Grav Force in Body/1(Euler)
  Rho/1 -> Alpha/Beta/2(Rho)
  NED(u)2b/1(Vb Corr) -> Alpha/Beta/1("Vx, Vy, Vz (Body)"), Vb Corr/1
  Body Frame F & M/2(M_b) -> Moments/1
  Gravitational Force/1 -> Get Grav Force in Body/2(Grav Force)
  Body Frame F & M/1(F_b) -> Sum/1
  Sum/1 -> Forces/1
  Alpha/Beta/3(qS) -> Body Frame F & M/3(qs)
  Alpha/Beta/4(Speed) -> Body Frame F & M/4(Airspeed), Airspeed/1
  "df, deg"/1 -> Body Frame F & M/8("df, deg")
  p,q,r/1 -> Body Frame F & M/9(p,q,r)
  Alpha/Beta/2("beta, deg") -> Body Frame F & M/2("Beta, deg")
  "dr, deg"/1 -> Body Frame F & M/7("dr, deg")
  da,deg/1 -> Body Frame F & M/6("da, deg")
  Alpha/Beta/1("alpha, deg") -> Body Frame F & M/1("Alpha, deg")
  "de, deg"/1 -> Body Frame F & M/5("de, deg")
  Wind e/1 -> Vair/2

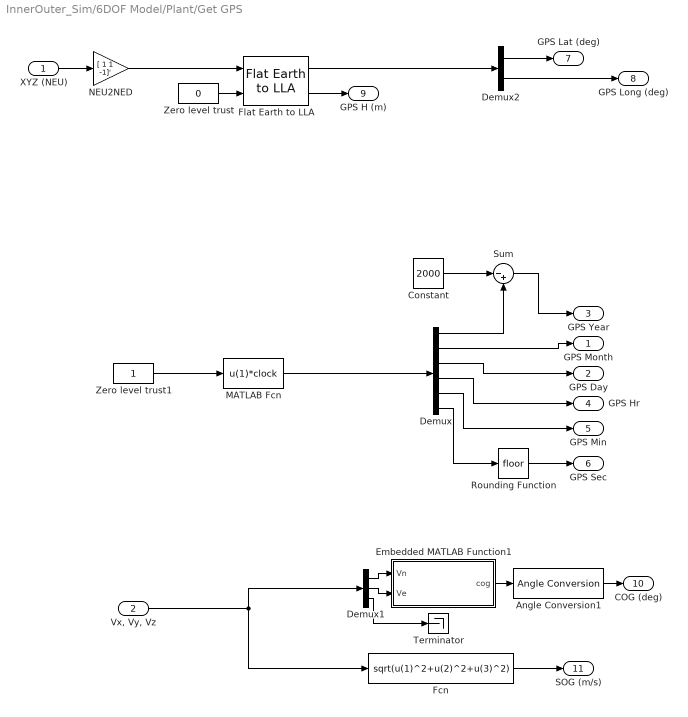
== system InnerOuter_Sim/6DOF Model/Plant/Get GPS ==
  XYZ (NEU) : Inport
  "Vx, Vy, Vz" : Inport  Port=2
  Angle Conversion1 : aerolibconvert2/Angle Conversion  SystemSampleTime=-1  IU=rad  OU=deg
  Constant : Constant  Value=2000
  Demux : Demux  Outputs=6
  Demux1 : Demux  Outputs=3
  Demux2 : Demux  Outputs=2
  Embedded MATLAB Function1 : Stateflow chart
  Fcn : Fcn  Expr=sqrt(u(1)^2+u(2)^2+u(3)^2)
  Flat Earth to LLA : aerolibtransform2/Flat Earth to LLA  SystemSampleTime=-1  units=Metric (MKS)  ptype=Earth (WGS84)  F=1/298.257223563  R=6378137  LL0=[37.0004768371582, -122.061897277832]  psi=0
  MATLAB Fcn : MATLABFcn  MATLABFcn=u(1)*clock  OutputSignalType=real  SampleTime=SampleT
  NEU2NED : Gain  Gain=[ 1 1 -1]'  SaturateOnIntegerOverflow=on
  Rounding Function : Rounding
  Sum : Sum  Inputs=|-+
  Terminator : Terminator
  Zero level trust : Constant  Value=0  SampleTime=SampleT
  Zero level trust1 : Constant  SampleTime=SampleT
  GPS Month : Outport
  GPS Day : Outport  Port=2
  GPS Year : Outport  Port=3
  GPS Hr : Outport  Port=4
  GPS Min : Outport  Port=5
  GPS Sec : Outport  Port=6
  GPS Lat (deg) : Outport  Port=7
  GPS Long (deg) : Outport  Port=8
  GPS H (m) : Outport  Port=9
  COG (deg) : Outport  Port=10
  SOG (m/s) : Outport  Port=11
  wires:
  NEU2NED/1 -> Flat Earth to LLA/1
  Zero level trust/1 -> Flat Earth to LLA/2
  XYZ (NEU)/1 -> NEU2NED/1
  Flat Earth to LLA/1 -> Demux2/1
  Flat Earth to LLA/2 -> GPS H (m)/1
  Zero level trust1/1 -> MATLAB Fcn/1
  MATLAB Fcn/1 -> Demux/1
  Demux/2 -> GPS Month/1
  Demux/3 -> GPS Day/1
  Demux/4 -> GPS Hr/1
  Demux/5 -> GPS Min/1
  Demux/6 -> Rounding Function/1
  Rounding Function/1 -> GPS Sec/1
  Demux2/1 -> GPS Lat (deg)/1
  Demux2/2 -> GPS Long (deg)/1
  Fcn/1 -> SOG (m/s)/1
  Demux1/1 -> Embedded MATLAB Function1/1(Vn)
  Demux1/2 -> Embedded MATLAB Function1/2(Ve)
  "Vx, Vy, Vz"/1 -> Demux1/1, Fcn/1
  Embedded MATLAB Function1/1(cog) -> Angle Conversion1/1
  Angle Conversion1/1 -> COG (deg)/1
  Demux/1 -> Sum/2
  Constant/1 -> Sum/1
  Sum/1 -> GPS Year/1
  Demux1/3 -> Terminator/1

== system InnerOuter_Sim/6DOF Model/Plant/ISA Atmosphere & Winds ==
  "X, Y, Z" : Inport
  Euler : Inport  Port=2
  Euler Angles to  Direction Cosine Matrix : aerolibtransform2/Euler Angles to  Direction Cosine Matrix  SystemSampleTime=-1
  Get Z : Selector  IndexOptions=Index vector (dialog)  Indices=[3]  OutputSizes=[(-2)]  InputPortWidth=3
  Horizontal Wind Model : aerolibwind2/Horizontal Wind Model  SystemSampleTime=-1  units=Metric (MKS)  Vw_source=Internal  Vwind=15  W_source=Internal  Wdeg=45
  ISA Atmosphere Model1 : aerolibatmos2/ISA Atmosphere Model  SystemSampleTime=-1  custom=off  g=9.80665  gamma=1.4  R=287.0531  L=0.0065  h_trop=11000  h_strat=20000  rho0=1.225  P0=101325  T0=288.15
  Scope : Scope
      settings: YMin=-2.5  YMax=2
  Terminator1 : Terminator
  Rho : Outport
  Wind : Outport  Port=2
  AirPressure (Pa) : Outport  Port=3
  OAT (K) : Outport  Port=4
  wires:
  "X, Y, Z"/1 -> Get Z/1
  Get Z/1 -> ISA Atmosphere Model1/1
  ISA Atmosphere Model1/4 -> Rho/1
  ISA Atmosphere Model1/1 -> OAT (K)/1
  ISA Atmosphere Model1/2 -> Terminator1/1
  ISA Atmosphere Model1/3 -> AirPressure (Pa)/1
  Euler Angles to  Direction Cosine Matrix/1 -> Horizontal Wind Model/1
  Euler/1 -> Euler Angles to  Direction Cosine Matrix/1
  Horizontal Wind Model/1 -> Scope/1, Wind/1

== system InnerOuter_Sim/6DOF Model/Plant/Magnetometer ==
  Euler : Inport
  LTP2B : dspmtrx3/Transpose  SystemSampleTime=-1  Hermitian=off  overflowFlag=off
  Mag Field in nT source:  http://www.ngdc.noaa.gov/geomagmodels/struts/calcIGRFWMM : Constant  Value=magField
  Product : Product  Multiplication=Matrix(*)  RndMeth=Zero
  RB2LTP : Subsystem
  "Mag, nT" : Outport
  wires:
  RB2LTP/1(Rot) -> LTP2B/1
  LTP2B/1 -> Product/1
  Mag Field in nT source:  http://www.ngdc.noaa.gov/geomagmodels/struts/calcIGRFWMM/1 -> Product/2
  Euler/1 -> RB2LTP/1(Euler)
  Product/1 -> "Mag, nT"/1

== system InnerOuter_Sim/6DOF Model/Plant/Wrap Around PSI1 ==
  Euler : Inport
  Compare To Zero : simulink/Logic and Bit Operations/Compare To Zero  SystemSampleTime=-1  relop=>=  LogicOutDataTypeMode=uint8  ZeroCross=off
  Logical Operator : Logic  Operator=NOT  AllPortsSameDT=off  OutDataTypeMode=Boolean
  Merge : Merge
  Mux2 : Mux  Inputs=2
  Negative Yaw : Subsystem
  Positive Yaw : Subsystem
  Selector1 : Selector  IndexOptions=Index vector (dialog)  Indices=[1 2]  OutputSizes=1  InputPortWidth=3
  Selector2 : Selector  IndexOptions=Index vector (dialog)  Indices=[3]  OutputSizes=1  InputPortWidth=3
  Euler-Wrapped : Outport
  wires:
  Euler/1 -> Selector2/1, Selector1/1
  Selector1/1 -> Mux2/1
  Mux2/1 -> Euler-Wrapped/1
  Selector2/1 -> Compare To Zero/1, Positive Yaw/1(yaw), Negative Yaw/1(yaw)
  Compare To Zero/1 -> Positive Yaw/Enable, Logical Operator/1
  Logical Operator/1 -> Negative Yaw/Enable
  Merge/1 -> Mux2/2
  Positive Yaw/1(yaw_wr) -> Merge/1
  Negative Yaw/1(yaw_wr) -> Merge/2

== system InnerOuter_Sim/Lateral Channel/psi_dot to Bank/Subsystem ==
  x : Inport
  C Function Call : dsPICdrivers/OTHERS/C Function Call  Tag=dsPIC_dsPIC_CFunctionCall  fctName='myAtan'  INPUT_SIZE=1  INPUT1=real64  INPUT2=--  INPUT3=--  OUTPUT_SIZE=1  OUTPUT1=real64  SampleTime=-1  InputType=[ 8 ]  OutputType=[ 8 ]  FctDeclaration=extern real64_T myAtan(real64_T u1);  FctCall=%y1 = myAtan(%u1);  OrderingInOutPopup=None
  Environment Controller : simulink/Signal Routing/Environment Controller  SystemSampleTime=-1
  Trigonometric Function : Trigonometry  Operator=atan
  atan(x) : Outport
  wires:
  x/1 -> C Function Call/1, Trigonometric Function/1
  Trigonometric Function/1 -> Environment Controller/1
  C Function Call/1 -> Environment Controller/2
  Environment Controller/1 -> atan(x)/1

== system InnerOuter_Sim/Longitudinal Channel/Airspeed Hold/Low_passed Time Derivative ==
  f(t) : Inport
  Add : Sum  OutScaling=2^-10
  Constant : Constant  Value=NDelay*TSample
  Divide : Product  Inputs=*/  OutScaling=2^-10
  Integer Delay : simulink/Discrete/Integer Delay  vinit=0.0  samptime=TSample  NumDelays=NDelay
  f_dot(t) : Outport
  wires:
  Divide/1 -> f_dot(t)/1
  Constant/1 -> Divide/2
  Integer Delay/1 -> Add/2
  f(t)/1 -> Integer Delay/1, Add/1
  Add/1 -> Divide/1

== system InnerOuter_Sim/6DOF Model/Plant/6-DOF EOM/Get Euler Dot ==
  p,q,r : Inport
  Euler : Inport  Port=2
  Mux1 : Mux  Inputs=[3 3]
  Mux2 : Mux  Inputs=3
  phidot : Fcn  Expr=u[1]+u[2]*sin(u[4])*tan(u[5])+u[3]*cos(u[4])*tan(u[5])
  psidot : Fcn  Expr=u[2]*sin(u[4])/cos(u[5])+u[3]*cos(u[4])/cos(u[5])
  thetadot : Fcn  Expr=u[2]*cos(u[4])-u[3]*sin(u[4])
  Euler_dot : Outport
  wires:
  Mux2/1 -> Euler_dot/1
  phidot/1 -> Mux2/1
  thetadot/1 -> Mux2/2
  psidot/1 -> Mux2/3
  Mux1/1 -> thetadot/1, phidot/1, psidot/1
  p,q,r/1 -> Mux1/1
  Euler/1 -> Mux1/2

== system InnerOuter_Sim/6DOF Model/Plant/6-DOF EOM/RB2LTP ==
  Euler : Inport
  11 : Fcn  Expr=cos(u[3])*cos(u[2])
  12 : Fcn  Expr=sin(u[3])*cos(u[2])
  13 : Fcn  Expr=-sin(u[2])
  21 : Fcn  Expr=cos(u[3])*sin(u[2])*sin(u[1])-sin(u[3])*cos(u[1])
  22 : Fcn  Expr=sin(u[3])*sin(u[2])*sin(u[1])+cos(u[3])*cos(u[1])
  23 : Fcn  Expr=cos(u[2])*sin(u[1])
  31 : Fcn  Expr=cos(u[3])*sin(u[2])*cos(u[1])+sin(u[3])*sin(u[1])
  32 : Fcn  Expr=sin(u[3])*sin(u[2])*cos(u[1])-cos(u[3])*sin(u[1])
  33 : Fcn  Expr=cos(u[2])*cos(u[1])
  Mux2 : Mux  Inputs=9
  Reshape : Reshape  OutputDimensionality=Customize  OutputDimensions=[3,3]
  Rot : Outport
  wires:
  33/1 -> Mux2/9
  32/1 -> Mux2/8
  31/1 -> Mux2/7
  23/1 -> Mux2/6
  22/1 -> Mux2/5
  21/1 -> Mux2/4
  13/1 -> Mux2/3
  12/1 -> Mux2/2
  11/1 -> Mux2/1
  Mux2/1 -> Reshape/1
  Euler/1 -> 11/1, 33/1, 32/1, 31/1, 23/1, 22/1, 21/1, 13/1, 12/1
  Reshape/1 -> Rot/1

== system InnerOuter_Sim/6DOF Model/Plant/6-DOF EOM/[V1,2,3,W1,2,3] ==
  note: V*dot =Inv(A){[F ; M] - SigmaAV*}
  "[F ; M]" : Inport
  Euler : Inport  Port=2
  V* : Inport  Port=3  PortDimensions=6
  A = [M ; J] : Subsystem
  Acc_meas : Product  Inputs=/*  Multiplication=Matrix(*)  SaturateOnIntegerOverflow=on  InputSameDT=on
  Demux : Demux  Outputs=[3;3]
  Get Grav Force in Body : Subsystem
  Gravitational Acc : Constant  Value=[0 0 -ISA_g]  VectorParams1D=off
  Selector3 : Selector  IndexOptions=Index vector (dialog)  Indices=1:3  OutputSizes=1  InputPortWidth=6
  Sigma : Subsystem
  Sigma*A : Product  Multiplication=Matrix(*)  SaturateOnIntegerOverflow=on  InputSameDT=on
  Sigma*A*V* : Product  Multiplication=Matrix(*)  SaturateOnIntegerOverflow=on  InputSameDT=on
  Sum1 : Sum  Inputs=+-|  SaturateOnIntegerOverflow=on  InputSameDT=on
  Sum2 : Sum  Inputs=++|  SaturateOnIntegerOverflow=on  InputSameDT=on
  Terminator1 : Terminator
  "V*dot " : Product  Inputs=/*  Multiplication=Matrix(*)  SaturateOnIntegerOverflow=on  InputSameDT=on
  "Acc_meas " : Outport
  V*dot : Outport  Port=2
  wires:
  Sum2/1 -> "Acc_meas "/1
  Get Grav Force in Body/1(Grav Force (Body)) -> Sum2/1
  Selector3/1 -> Sum2/2
  Euler/1 -> Get Grav Force in Body/1(Euler)
  Gravitational Acc/1 -> Get Grav Force in Body/2(Grav Force)
  Acc_meas/1 -> Selector3/1
  Sigma*A/1 -> Sigma*A*V*/1
  "V*dot "/1 -> V*dot/1
  V*/1 -> Demux/1, Sigma*A*V*/2
  Demux/2 -> Sigma/1(pqr)
  Sigma*A*V*/1 -> Sum1/2
  "[F ; M]"/1 -> Acc_meas/2, Sum1/1
  Sigma/1(Sigma) -> Sigma*A/1
  Demux/1 -> Terminator1/1
  A = [M ; J]/1(A Matrix) -> Acc_meas/1, "V*dot "/1, Sigma*A/2
  Sum1/1 -> "V*dot "/2
